simulink library "LiveParts"  (Simulink 8.7)
settings: Solver=ode45  StartTime=0.0  StopTime=10.0  RelTol=1e-3
undefined symbols (not defined in the file): a, unspecifiedConstant, unspecifiedMatrix
settings Model: Creator=christopher.wipf  LastModifiedBy=controls

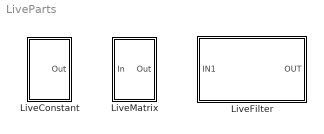
== system LiveParts ==
  LiveConstant : Subsystem  Tag=LiveConstant  mask{K=unspecifiedConstant, chan='unspecifiedChannel'}
      mask prompts: K "Constant"; chan "Channel"
      settings: AttributesFormatString=%<Tag>
      mask Display: disp(K)
  LiveFilter : Subsystem  Tag=LiveFilter  mask{par=a, prefix='unspecifiedChannel', site='unspecifiedSite', feModel='unspecifiedModel', fmName='unspecifiedName', flexTf=on, viewGui=off}
      mask prompts: par "FM parameter struct"; prefix "Channel prefix"; feModel "FE model name"; fmName "FM name"; flexTf "Use FlexTf"; viewGui "Click to view/edit config"
      mask init:
      | if flexTf
      |     set_param([gcb '/FM1'], 'Description', ['FlexTf: par.fm1frd']);
      |     set_param([gcb '/FM2'], 'Description', ['FlexTf: par.fm2frd']);
      |     set_param([gcb '/FM3'], 'Description', ['FlexTf: par.fm3frd']);
      |     set_param([gcb '/FM4'], 'Description', ['FlexTf: par.fm4frd']);
      |     set_param([gcb '/FM5'], 'Description', ['FlexTf: par.fm5frd']);
      |     set_param([gcb '/FM6'], 'Description', ['FlexTf: par.fm6frd']);
      |     set_param([gcb '/FM7'], 'Description', ['FlexTf: par.fm7frd']);
      |     set_param([gcb '/FM8'], 'Description', ['FlexTf: par.fm8frd']);
      |     set_param([gcb '/FM9'], 'Description', ['FlexTf: par.fm9frd']);
      |     set_param([gcb '/FM10'], 'Description', ['FlexTf: par.fm10frd']);
      | else
      |     set_param([gcb '/FM1'], 'Description', '');
      |     set_param([gcb '/FM2'], 'Description', '');
      |     set_param([gcb '/FM3'], 'Description', '');
      |     set_param([gcb '/FM4'], 'Description', '');
      |     set_param([gcb '/FM5'], 'Description', '');
      |     set_param([gcb '/FM6'], 'Description', '');
      |     set_param([gcb '/FM7'], 'Description', '');
      |     set_param([gcb '/FM8'], 'Description', '');
      |     set_param([gcb '/FM9'], 'Description', '');
      |     set_param([gcb '/FM10'], 'Description', '');
      | end
      settings: AttributesFormatString=%<Tag>
      mask Callback viewGui: viewLiveFilter(gcb);
      mask Display:
      | if isstruct(par) && isfield(par, 'fm1')
      |     if flexTf
      |         disp([get_param(gcb, 'par') char(10) 'FlexTf']);
      |     else
      |         disp(get_param(gcb, 'par'));
      |     end
      | else
      |     disp('???')
      | end
  LiveMatrix : Subsystem  Tag=LiveMatrix  mask{M=unspecifiedMatrix, prefix='unspecifiedChannel', firstRow=1, firstCol=1, lastRow=1, lastCol=1}
      mask prompts: M "Matrix"; prefix "Channel prefix"; firstRow "First row"; firstCol "First column"; lastRow "Last row"; lastCol "Last column"
      settings: AttributesFormatString=%<Tag>
      mask Display: disp([get_param(gcb, 'M') '*u']);

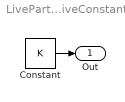
== system LiveParts/LiveConstant ==
  Constant : Constant  Value=K
  Out : Outport
  wires:
  Constant/1 -> Out/1

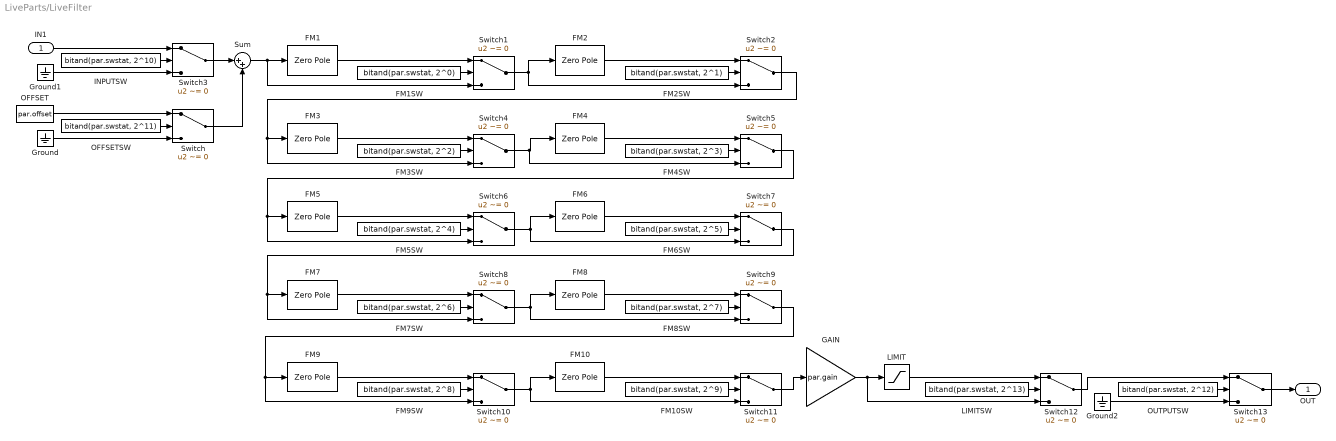
== system LiveParts/LiveFilter ==
  IN1 : Inport
  FM1 : ZeroPole  Description=FlexTf: par.fm1frd  Zeros=par.fm1.z{1}  Poles=par.fm1.p{1}  Gain=par.fm1.k
  FM10 : ZeroPole  Description=FlexTf: par.fm10frd  Zeros=par.fm10.z{1}  Poles=par.fm10.p{1}  Gain=par.fm10.k
  FM10SW : Constant  Value=bitand(par.swstat, 2^9)
  FM1SW : Constant  Value=bitand(par.swstat, 2^0)
  FM2 : ZeroPole  Description=FlexTf: par.fm2frd  Zeros=par.fm2.z{1}  Poles=par.fm2.p{1}  Gain=par.fm2.k
  FM2SW : Constant  Value=bitand(par.swstat, 2^1)
  FM3 : ZeroPole  Description=FlexTf: par.fm3frd  Zeros=par.fm3.z{1}  Poles=par.fm3.p{1}  Gain=par.fm3.k
  FM3SW : Constant  Value=bitand(par.swstat, 2^2)
  FM4 : ZeroPole  Description=FlexTf: par.fm4frd  Zeros=par.fm4.z{1}  Poles=par.fm4.p{1}  Gain=par.fm4.k
  FM4SW : Constant  Value=bitand(par.swstat, 2^3)
  FM5 : ZeroPole  Description=FlexTf: par.fm5frd  Zeros=par.fm5.z{1}  Poles=par.fm5.p{1}  Gain=par.fm5.k
  FM5SW : Constant  Value=bitand(par.swstat, 2^4)
  FM6 : ZeroPole  Description=FlexTf: par.fm6frd  Zeros=par.fm6.z{1}  Poles=par.fm6.p{1}  Gain=par.fm6.k
  FM6SW : Constant  Value=bitand(par.swstat, 2^5)
  FM7 : ZeroPole  Description=FlexTf: par.fm7frd  Zeros=par.fm7.z{1}  Poles=par.fm7.p{1}  Gain=par.fm7.k
  FM7SW : Constant  Value=bitand(par.swstat, 2^6)
  FM8 : ZeroPole  Description=FlexTf: par.fm8frd  Zeros=par.fm8.z{1}  Poles=par.fm8.p{1}  Gain=par.fm8.k
  FM8SW : Constant  Value=bitand(par.swstat, 2^7)
  FM9 : ZeroPole  Description=FlexTf: par.fm9frd  Zeros=par.fm9.z{1}  Poles=par.fm9.p{1}  Gain=par.fm9.k
  FM9SW : Constant  Value=bitand(par.swstat, 2^8)
  GAIN : Gain  Gain=par.gain
  Ground : Ground
  Ground1 : Ground
  Ground2 : Ground
  INPUTSW : Constant  Value=bitand(par.swstat, 2^10)
  LIMIT : Saturate  UpperLimit=par.limit  LowerLimit=-par.limit
  LIMITSW : Constant  Value=bitand(par.swstat, 2^13)
  OFFSET : Constant  Value=par.offset
  OFFSETSW : Constant  Value=bitand(par.swstat, 2^11)
  OUTPUTSW : Constant  Value=bitand(par.swstat, 2^12)
  Sum : Sum  Inputs=|++
  Switch{,1..13} (14 alike) : Switch  Criteria=u2 ~= 0
  OUT : Outport
  wires:
  GAIN/1 -> Switch12/3, LIMIT/1
  Sum/1 -> FM1/1, Switch1/3
  OFFSET/1 -> Switch/1
  Ground/1 -> Switch/3
  OFFSETSW/1 -> Switch/2
  Switch1/1 -> FM2/1, Switch2/3
  FM1/1 -> Switch1/1
  FM1SW/1 -> Switch1/2
  FM2/1 -> Switch2/1
  FM2SW/1 -> Switch2/2
  Switch2/1 -> FM3/1, Switch4/3
  INPUTSW/1 -> Switch3/2
  Ground1/1 -> Switch3/3
  IN1/1 -> Switch3/1
  FM3/1 -> Switch4/1
  Switch4/1 -> FM4/1, Switch5/3
  FM4/1 -> Switch5/1
  FM4SW/1 -> Switch5/2
  FM3SW/1 -> Switch4/2
  Switch5/1 -> FM5/1, Switch6/3
  FM5/1 -> Switch6/1
  Switch6/1 -> FM6/1, Switch7/3
  FM5SW/1 -> Switch6/2
  FM6/1 -> Switch7/1
  Switch7/1 -> FM7/1, Switch8/3
  FM6SW/1 -> Switch7/2
  FM7/1 -> Switch8/1
  FM7SW/1 -> Switch8/2
  Switch8/1 -> FM8/1, Switch9/3
  FM8/1 -> Switch9/1
  FM8SW/1 -> Switch9/2
  Switch9/1 -> FM9/1, Switch10/3
  FM9/1 -> Switch10/1
  FM9SW/1 -> Switch10/2
  Switch10/1 -> FM10/1, Switch11/3
  FM10/1 -> Switch11/1
  FM10SW/1 -> Switch11/2
  Switch11/1 -> GAIN/1
  LIMIT/1 -> Switch12/1
  LIMITSW/1 -> Switch12/2
  Switch12/1 -> Switch13/1
  Ground2/1 -> Switch13/3
  OUTPUTSW/1 -> Switch13/2
  Switch13/1 -> OUT/1
  Switch3/1 -> Sum/1
  Switch/1 -> Sum/2

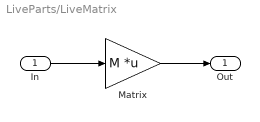
== system LiveParts/LiveMatrix ==
  In : Inport
  Matrix : Gain  Gain=M  Multiplication=Matrix(K*u)
  Out : Outport
  wires:
  In/1 -> Matrix/1
  Matrix/1 -> Out/1
